simulink model "AdaptiveControl_jointSpace_AfterRedunElimi_1"  (R2020a)
settings: Solver=FixedStepDiscrete  StartTime=0.0  StopTime=Inf  FixedStep=0.001  RelTol=1e-3  EnableMultiTasking=on
values from neighbouring files (symbols this model uses):
  qr = [0 9.85590088848e-08 3.94236035539e-07 8.87031079963e-07 1.57694414216e-06 2.46397522212e-06 3.54812431985e-06 4.82939143535e-06 6.30777656863e-06 7.98327971967e-06 9.85590088848e-06 1.19256400751e-05 ... (188496 elements, 62832x3)]    [qr_62s.mat]
undefined symbols (not defined in the file or in its folder): DiscIntNeverNeededParam
libraries: slrealtimeethercatlib x27
settings Model: xpc_rtwmakecfg_data=_xpcethercatlib_  SimulationMode=external  Creator=hung  LastModifiedBy=Hung
settings SolverCC: ConcurrentTasks=on  AutoInsertRateTranBlk=on  InsertRTBMode=Never (minimum delay)
settings DataIOCC: SaveFormat=StructureWithTime  SaveState=on  SignalLoggingName=logsOut
settings OptimizationCC: BlockReduction=off  BooleanDataType=off  OptimizeBlockIOStorage=off  BufferReuse=off  GlobalBufferReuse=off  ExpressionFolding=off  LocalBlockOutputs=off  InitFltsAndDblsToZero=on  OptimizeDataStoreBuffers=off  BusAssignmentInplaceUpdate=off
settings DebuggingCC: SaveWithParameterizedLinksMsg=none  UnderspecifiedInitializationDetection=Classic  MergeDetectMultiDrivingBlocksExec=none  CheckExecutionContextPreStartOutputMsg=on  SignalResolutionControl=TryResolveAllWithWarning  SFUnexpectedBacktrackingDiag=warning  SFNoUnconditionalDefaultTransitionDiag=warning  SFExecutionAtInitializationDiag=none  UnderSpecifiedDimensionMsg=warning  ArithmeticOperatorsInVariantConditions=warning
settings HardwareCC: ProdBitPerPointer=32  ProdBitPerSizeT=32  ProdBitPerPtrDiffT=32  ProdLargestAtomicFloat=None  ProdWordSize=32  ProdLongLongMode=on  ProdHWDeviceType=Generic->32-bit x86 compatible
settings ModelReferenceCC: PropagateSignalLabelsOutOfModel=off
settings SFSimCC: SimUseLocalCustomCode=off
settings RTWCC: Description=Simulink Real-Time  SystemTargetFile=slrt.tlc  TemplateMakefile=slrt_default_tmf  RTWUseLocalCustomCode=off  CodeExecutionProfiling=on  RTWCompilerOptimization=on
settings CodeAppCC: StateflowObjectComments=on
settings SimulinkRealTimeCC: SupportVariableSizeSignals=on  RL32LogTETModifier=off  xPCConcurrentTasks=on
settings ConfigComp: CovMetricSettings=dw  CovSaveCumulativeToWorkspaceVar=on  CovSaveSingleToWorkspaceVar=on  CovExternalEMLEnable=off  CovSFcnEnable=off

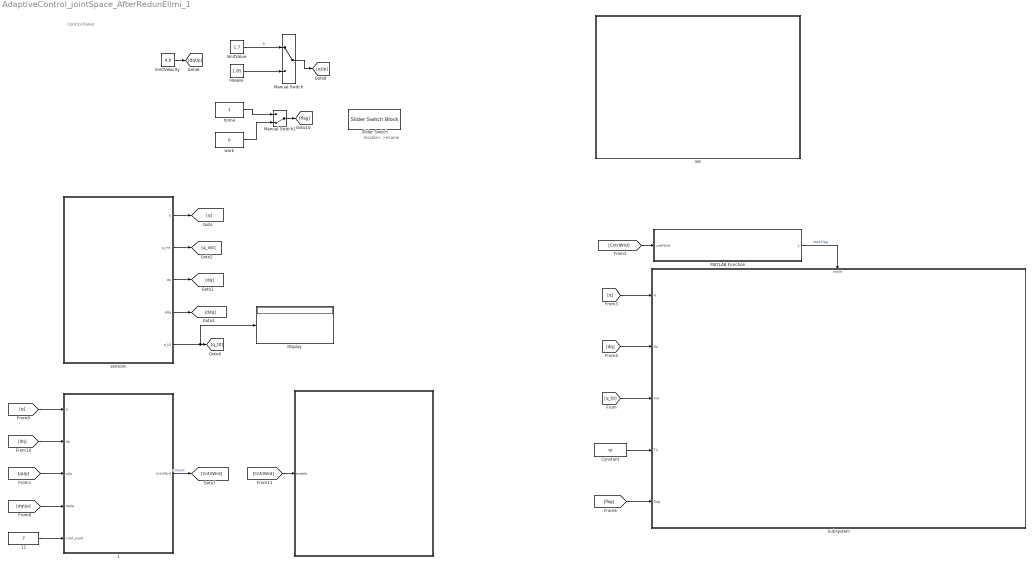
== system AdaptiveControl_jointSpace_AfterRedunElimi_1 ==
  note: Control Panel
  note: disable< >enable
  "  " : Subsystem
  1 : MATLAB Function  TreatAsAtomicUnit=on
  11 : Constant  Value=7
  Constant : Constant  Value=qr
  Display : Display
  MATLAB Function : MATLAB Function  TreatAsAtomicUnit=on
  Manual Switch : ManualSwitch
  Manual Switch1 : ManualSwitch  CurrentSetting=0
  Slider Switch : SliderSwitchBlock  LabelPosition=Hide
      settings: Values={{'Off', 'On'}, [7 15]}
  Subsystem : Subsystem
  home : Constant
  init : Subsystem
  limitValue : Constant  Value=1.7
  limitVelocity : Constant  Value=4.0
  release : Constant  Value=1.85
  sensore : Subsystem
  work : Constant  Value=0
  wires:
  ? -> ?
  sensore/1(q) -> [q]
  sensore/2(q_init) -> [q_init]
  sensore/3(dq) -> [dq]
  sensore/4(ddq) -> [ddq]
  1/1(CntrlWrd) -> [CntrlWrd]  "cntwrd"
  11/1 -> 1/5(cntrl_word)
  [dq] -> 1/2(dq)
  [q] -> 1/1(q)
  [CntrlWrd] -> "  "/1(enable)
  [qUp] -> 1/3(qUp)
  [dqUp] -> 1/4(dqUp)
  limitVelocity/1 -> [dqUp]
  limitValue/1 -> Manual Switch/1  "9"
  release/1 -> Manual Switch/2
  Manual Switch/1 -> [qUp]
  MATLAB Function/1(y) -> Subsystem/Enable  "startFlag"
  [CntrlWrd] -> MATLAB Function/1(cntrlWrd)
  sensore/5(q_t0) -> Display/1, [q_t0]
  Constant/1 -> Subsystem/4(Trj)
  work/1 -> Manual Switch1/2
  home/1 -> Manual Switch1/1
  [flag] -> Subsystem/5(flag)
  Manual Switch1/1 -> [flag]
  [q_t0] -> Subsystem/3(In3)
  [q] -> Subsystem/1(q)
  [dq] -> Subsystem/2(dq)

== system AdaptiveControl_jointSpace_AfterRedunElimi_1/   ==
  note: Contrword_setting
  enable : Inport
  Data Type Conversion : DataTypeConversion  OutDataTypeStr=uint16
  Enabled Subsystem : Subsystem  TreatAsAtomicUnit=on
  Step1 : Step  Time=5.5  SampleTime=0
  controlword_transmit : Subsystem
  wires:
  enable/1 -> Enabled Subsystem/1(In1)
  Step1/1 -> Enabled Subsystem/Enable
  Enabled Subsystem/1(ctrword) -> Data Type Conversion/1  "contrlw"
  Data Type Conversion/1 -> controlword_transmit/1(In2), controlword_transmit/2(In4), controlword_transmit/3(In6)

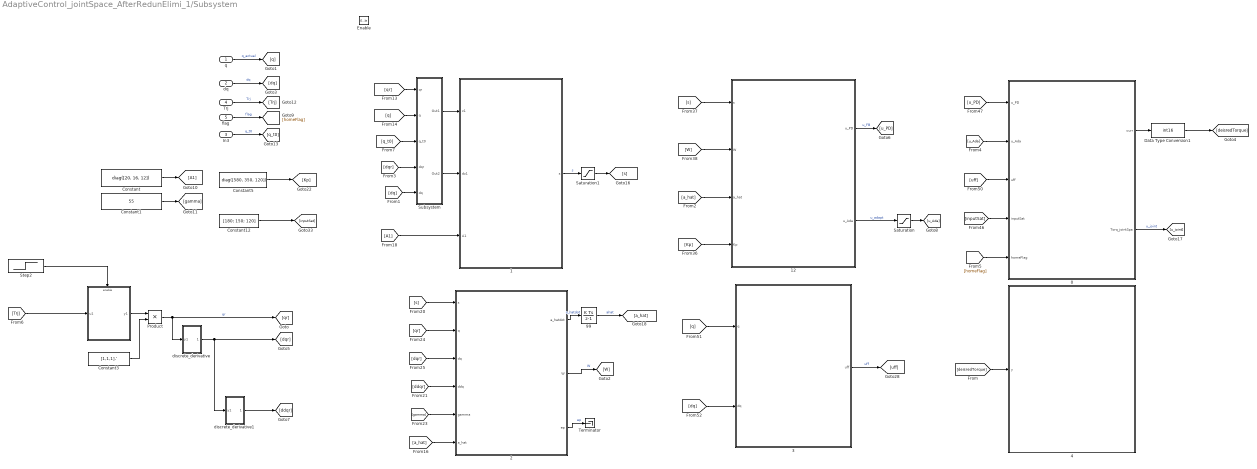
== system AdaptiveControl_jointSpace_AfterRedunElimi_1/Subsystem ==
  q : Inport
  dq : Inport  Port=2
  In3 : Inport  Port=3
  Trj : Inport  Port=4
  flag : Inport  Port=5
  Enable : EnablePort
  " " : Subsystem  TreatAsAtomicUnit=on
  0 : MATLAB Function  TreatAsAtomicUnit=on
  1 : MATLAB Function  TreatAsAtomicUnit=on
  12 : MATLAB Function  TreatAsAtomicUnit=on
  2 : MATLAB Function  TreatAsAtomicUnit=on
  3 : MATLAB Function  TreatAsAtomicUnit=on
  4 : Subsystem
  99 : DiscreteIntegrator  InitialCondition=zeros(12,1)  SampleTime=-1  ICPrevOutput=DiscIntNeverNeededParam  ICPrevScaledInput=DiscIntNeverNeededParam
  Constant : Constant  Value=diag([20, 16, 12])  VectorParams1D=off
  Constant1 : Constant  Value=55  VectorParams1D=off
  Constant12 : Constant  Value=[180; 150; 120]  VectorParams1D=off
  Constant3 : Constant  Value=[1,1,1].'  VectorParams1D=off
  Constant5 : Constant  Value=diag([580, 350, 120])  VectorParams1D=off
  Data Type Conversion1 : DataTypeConversion  OutDataTypeStr=int16
  Product : Product
  Saturation : Saturate  UpperLimit=180  LowerLimit=-180
  Saturation1 : Saturate  UpperLimit=1  LowerLimit=-1
  Step2 : Step  Time=2  SampleTime=0
  Subsystem : Subsystem
  Terminator : Terminator
  discrete_derivative : Subsystem
  discrete_derivative1 : Subsystem
  wires:
  Constant1/1 -> [gamma]
  2/1(a_hatdot) -> 99/1  "a_hatdot"
  Constant/1 -> [A1]
  [s] -> 12/1(s)
  [gamma] -> 2/5(gamma)
  0/1(curr) -> Data Type Conversion1/1
  [ddqr] -> 2/4(ddq)
  Data Type Conversion1/1 -> [deisredTorque]
  [qr] -> 2/2(q)
  [W] -> 12/2(W)
  [inputSat] -> 0/4(inputSat)
  [u_PD] -> 0/1(u_PD)
  3/1(uff) -> [uff]  "uff"
  [dqr] -> 2/3(dq)
  Constant5/1 -> [Kp]
  [Kp] -> 12/4(Kp)
  Constant12/1 -> [inputSat]
  [dq] -> 3/2(dq)
  1/1(s) -> Saturation1/1  "s"
  [A1] -> 1/3(A1)
  [q] -> 3/1(q)
  [deisredTorque] -> 4/1(y)
  q/1 -> [q]  "q_actual"
  dq/1 -> [dq]  "dq"
  [q] -> Subsystem/2(q)
  Subsystem/1(Out1) -> 1/1(z1)
  Subsystem/2(Out2) -> 1/2(dz1)
  99/1 -> [a_hat]  "ahat"
  [dq] -> Subsystem/5(dq)
  0/2(Torq_jointSpa) -> [u_joint]  "u_joint"
  2/2(W) -> [W]  "W"
  [a_hat] -> 12/3(a_hat)
  [uff] -> 0/3(uff)
  Product/1 -> discrete_derivative/1(y1), [qr]  "qr"
  Step2/1 -> " "/Enable
  [dqr] -> Subsystem/4(dqr)
  discrete_derivative/1(Out1) -> discrete_derivative1/1(y1), [dqr]
  discrete_derivative1/1(Out1) -> [ddqr]
  [qr] -> Subsystem/1(qr)
  12/1(u_PD) -> [u_PD]  "u_FB"
  12/2(u_Ada) -> Saturation/1  "u_adapt"
  [u_Ada] -> 0/2(u_Ada)
  [homeFlag] -> 0/5(homeFlag)
  Trj/1 -> [Trj]  "Trj"
  flag/1 -> [homeFlag]  "flag"
  In3/1 -> [q_t0]  "q_t0"
  [q_t0] -> Subsystem/3(q_t0)
  [a_hat] -> 2/6(a_hat)
  2/3(ep) -> Terminator/1  "ep"
  [Trj] -> " "/1(u1)
  " "/1(y1) -> Product/1
  Constant3/1 -> Product/2
  Saturation/1 -> [u_Ada]
  [s] -> 2/1(s)
  Saturation1/1 -> [s]

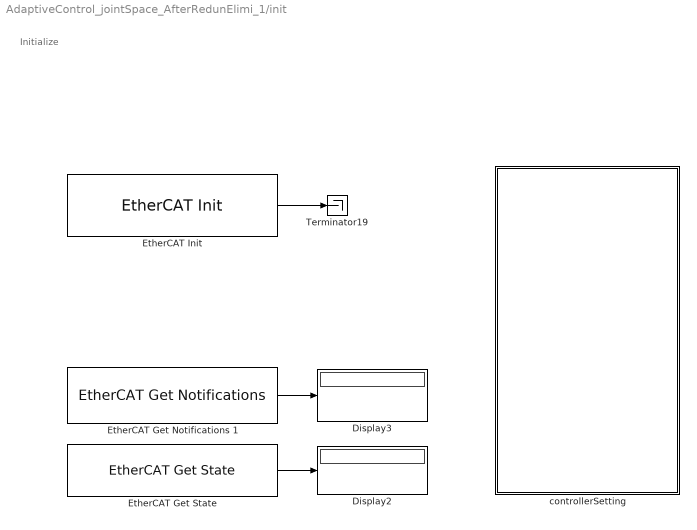
== system AdaptiveControl_jointSpace_AfterRedunElimi_1/init ==
  note: Initialize
  Display2 : Display
      settings: Format=hex (Stored Integer)
  Display3 : Display
      settings: Format=hex (Stored Integer)
  EtherCAT Get Notifications 1 : slrealtimeethercatlib/EtherCAT Get Notifications  device_id=0  sample_time=.001
  "EtherCAT Get State  " : slrealtimeethercatlib/EtherCAT Get State  device_id=0  sample_time=0
  "EtherCAT Init " : slrealtimeethercatlib/EtherCAT Init  Priority=0  config_file=E:\hhz_SRStest\EfficientModeling_Experimment\allJioints\eni8.xml  device_id=0  pci_bus=0  pci_slot=0  pci_function=0  portnum=1  initstate=2  dctuning=0  enaDebug=0  enaDC=on  errLink=off  masterDbg=off  stateChgDbg=off  baseClock=off  masterCfg=off  logFile='c:\dbglog.txt'  sample_time=0.001000  DCMode=2
  Terminator19 : Terminator
  controllerSetting : Subsystem
  wires:
  EtherCAT Get Notifications 1/1 -> Display3/1
  "EtherCAT Get State  "/1 -> Display2/1
  "EtherCAT Init "/1 -> Terminator19/1

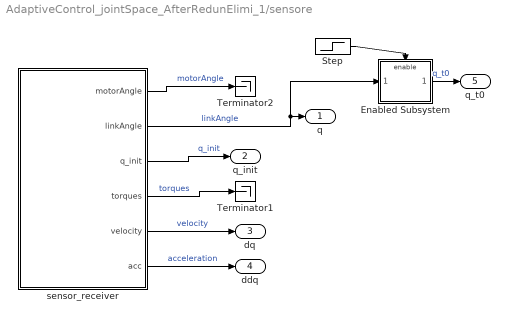
== system AdaptiveControl_jointSpace_AfterRedunElimi_1/sensore ==
  Enabled Subsystem : Subsystem  TreatAsAtomicUnit=on
  Step : Step  Time=6  Before=1  After=0  SampleTime=0
  Terminator1 : Terminator
  Terminator2 : Terminator
  sensor_receiver : Subsystem
  q : Outport
  q_init : Outport  Port=2
  dq : Outport  Port=3
  ddq : Outport  Port=4
  q_t0 : Outport  Port=5
  wires:
  sensor_receiver/3(q_init) -> q_init/1  "q_init"
  sensor_receiver/4(torques) -> Terminator1/1  "torques"
  sensor_receiver/1(motorAngle) -> Terminator2/1  "motorAngle"
  sensor_receiver/5(velocity) -> dq/1  "velocity"
  sensor_receiver/2(linkAngle) -> Enabled Subsystem/1(linkAngle), q/1  "linkAngle"
  sensor_receiver/6(acc) -> ddq/1  "acceleration"
  Step/1 -> Enabled Subsystem/Enable
  Enabled Subsystem/1(Out1) -> q_t0/1  "q_t0"

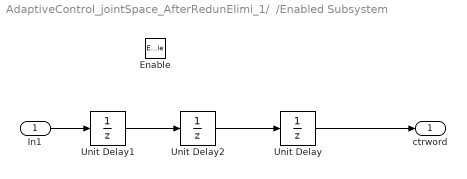
== system AdaptiveControl_jointSpace_AfterRedunElimi_1/  /Enabled Subsystem ==
  In1 : Inport
  Enable : EnablePort
  Unit Delay : UnitDelay  SampleTime=-1  HasFrameUpgradeWarning=on
  Unit Delay1 : UnitDelay  InitialCondition=7  SampleTime=-1  HasFrameUpgradeWarning=on
  Unit Delay2 : UnitDelay  InitialCondition=6  SampleTime=-1  HasFrameUpgradeWarning=on
  ctrword : Outport
  wires:
  In1/1 -> Unit Delay1/1
  Unit Delay1/1 -> Unit Delay2/1
  Unit Delay2/1 -> Unit Delay/1
  Unit Delay/1 -> ctrword/1

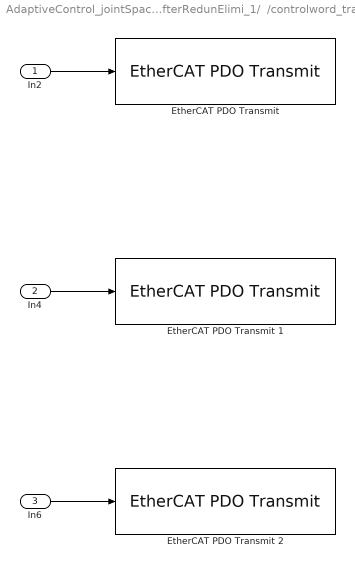
== system AdaptiveControl_jointSpace_AfterRedunElimi_1/  /controlword_transmit ==
  In2 : Inport
  In4 : Inport  Port=2
  In6 : Inport  Port=3
  "EtherCAT PDO Transmit " : slrealtimeethercatlib/EtherCAT PDO Transmit  Priority=3  sig_name=Slave_1002 [Elmo Drive ].Outputs.ControlWord  sig_offset=144  sig_type=uint16  type_size=16  sig_dim=1  device_id=0  sample_time=0.001000
  EtherCAT PDO Transmit 1 : slrealtimeethercatlib/EtherCAT PDO Transmit  Priority=3  sig_name=Slave_1004 [Elmo Drive ].Outputs.ControlWord  sig_offset=432  sig_type=uint16  type_size=16  sig_dim=1  device_id=0  sample_time=0.001000
  EtherCAT PDO Transmit 2 : slrealtimeethercatlib/EtherCAT PDO Transmit  Priority=3  sig_name=Slave_1006 [Elmo Drive ].Outputs.ControlWord  sig_offset=720  sig_type=uint16  type_size=16  sig_dim=1  device_id=0  sample_time=0.001000
  wires:
  In4/1 -> EtherCAT PDO Transmit 1/1
  In2/1 -> "EtherCAT PDO Transmit "/1
  In6/1 -> EtherCAT PDO Transmit 2/1

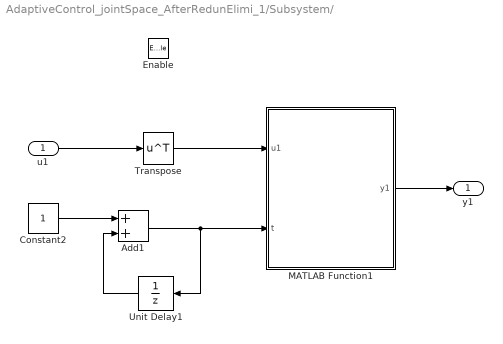
== system AdaptiveControl_jointSpace_AfterRedunElimi_1/Subsystem/  ==
  u1 : Inport
  Enable : EnablePort  StatesWhenEnabling=reset
  Add1 : Sum
  Constant2 : Constant
  MATLAB Function1 : MATLAB Function  TreatAsAtomicUnit=on
  Transpose : Math  Operator=transpose  SaturateOnIntegerOverflow=on
  Unit Delay1 : UnitDelay  SampleTime=-1  HasFrameUpgradeWarning=on
  y1 : Outport
  wires:
  MATLAB Function1/1(y1) -> y1/1
  Constant2/1 -> Add1/1
  Unit Delay1/1 -> Add1/2
  u1/1 -> Transpose/1
  Add1/1 -> Unit Delay1/1, MATLAB Function1/2(t)
  Transpose/1 -> MATLAB Function1/1(u1)

== system AdaptiveControl_jointSpace_AfterRedunElimi_1/Subsystem/4 ==
  y : Inport
  Demux : Demux  Outputs=3
  transmit : Subsystem
  wires:
  y/1 -> Demux/1
  Demux/3 -> transmit/3(theta6)
  Demux/2 -> transmit/2(theta4)
  Demux/1 -> transmit/1(theta2)

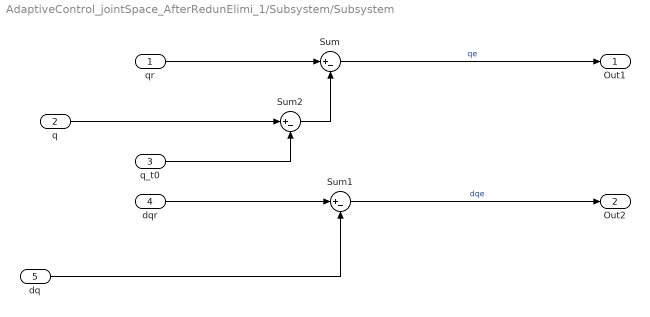
== system AdaptiveControl_jointSpace_AfterRedunElimi_1/Subsystem/Subsystem ==
  qr : Inport
  q : Inport  Port=2
  q_t0 : Inport  Port=3
  dqr : Inport  Port=4
  dq : Inport  Port=5
  Sum : Sum  Inputs=|+-
  Sum1 : Sum  Inputs=|+-
  Sum2 : Sum  Inputs=|+-
  Out1 : Outport
  Out2 : Outport  Port=2
  wires:
  qr/1 -> Sum/1
  Sum/1 -> Out1/1  "qe"
  dqr/1 -> Sum1/1
  dq/1 -> Sum1/2
  Sum1/1 -> Out2/1  "dqe"
  q/1 -> Sum2/1
  Sum2/1 -> Sum/2
  q_t0/1 -> Sum2/2

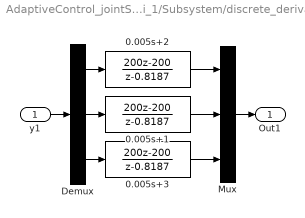
== system AdaptiveControl_jointSpace_AfterRedunElimi_1/Subsystem/discrete_derivative ==
  y1 : Inport
  0.005s+1 : DiscreteTransferFcn  Numerator=[200, -200]  Denominator=[1 -0.8187]
  0.005s+2 : DiscreteTransferFcn  Numerator=[200, -200]  Denominator=[1 -0.8187]
  0.005s+3 : DiscreteTransferFcn  Numerator=[200, -200]  Denominator=[1 -0.8187]
  Demux : Demux  Outputs=3
  Mux : Mux  Inputs=3
  Out1 : Outport
  wires:
  0.005s+1/1 -> Mux/2
  Mux/1 -> Out1/1
  Demux/2 -> 0.005s+1/1
  y1/1 -> Demux/1
  0.005s+2/1 -> Mux/1
  Demux/1 -> 0.005s+2/1
  0.005s+3/1 -> Mux/3
  Demux/3 -> 0.005s+3/1

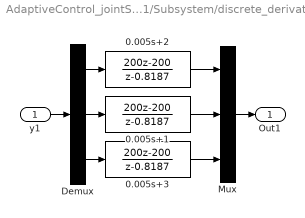
== system AdaptiveControl_jointSpace_AfterRedunElimi_1/Subsystem/discrete_derivative1 ==
  y1 : Inport
  0.005s+1 : DiscreteTransferFcn  Numerator=[200, -200]  Denominator=[1 -0.8187]
  0.005s+2 : DiscreteTransferFcn  Numerator=[200, -200]  Denominator=[1 -0.8187]
  0.005s+3 : DiscreteTransferFcn  Numerator=[200, -200]  Denominator=[1 -0.8187]
  Demux : Demux  Outputs=3
  Mux : Mux  Inputs=3
  Out1 : Outport
  wires:
  0.005s+1/1 -> Mux/2
  Mux/1 -> Out1/1
  Demux/2 -> 0.005s+1/1
  y1/1 -> Demux/1
  0.005s+2/1 -> Mux/1
  Demux/1 -> 0.005s+2/1
  0.005s+3/1 -> Mux/3
  Demux/3 -> 0.005s+3/1

== system AdaptiveControl_jointSpace_AfterRedunElimi_1/init/controllerSetting ==
  Data Type Conversion2 : DataTypeConversion  OutDataTypeStr=int8
  change_mode : Step  Time=5.3  After=10  SampleTime=0
  contr_loop_Mode : Subsystem
  wires:
  change_mode/1 -> Data Type Conversion2/1
  Data Type Conversion2/1 -> contr_loop_Mode/1(In1)

== system AdaptiveControl_jointSpace_AfterRedunElimi_1/sensore/Enabled Subsystem ==
  linkAngle : Inport
  Enable : EnablePort
  Out1 : Outport
  wires:
  linkAngle/1 -> Out1/1

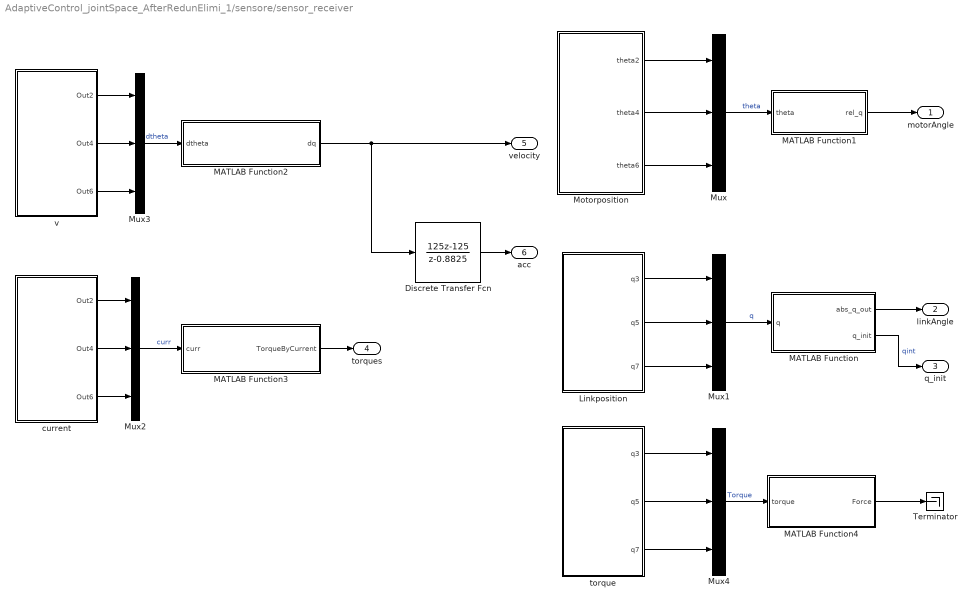
== system AdaptiveControl_jointSpace_AfterRedunElimi_1/sensore/sensor_receiver ==
  Discrete Transfer Fcn : DiscreteTransferFcn  Numerator=[125 -125]  Denominator=[1 -0.8825]
  Linkposition : Subsystem
  MATLAB Function : MATLAB Function  TreatAsAtomicUnit=on
  MATLAB Function1 : MATLAB Function  TreatAsAtomicUnit=on
  MATLAB Function2 : MATLAB Function  TreatAsAtomicUnit=on
  MATLAB Function3 : MATLAB Function  TreatAsAtomicUnit=on
  MATLAB Function4 : MATLAB Function  TreatAsAtomicUnit=on
  Motorposition : Subsystem
  Mux{,1..4} (5 alike) : Mux  Inputs=3
  Terminator : Terminator
  current : Subsystem
  torque : Subsystem
  v : Subsystem
  motorAngle : Outport
  linkAngle : Outport  Port=2
  q_init : Outport  Port=3
  torques : Outport  Port=4
  velocity : Outport  Port=5
  acc : Outport  Port=6
  wires:
  Mux/1 -> MATLAB Function1/1(theta)  "theta"
  MATLAB Function/2(q_init) -> q_init/1  "qint"
  Mux1/1 -> MATLAB Function/1(q)  "q"
  Mux3/1 -> MATLAB Function2/1(dtheta)  "dtheta"
  Linkposition/1(q3) -> Mux1/1
  Linkposition/2(q5) -> Mux1/2
  Linkposition/3(q7) -> Mux1/3
  Motorposition/1(theta2) -> Mux/1
  Motorposition/3(theta6) -> Mux/3
  Motorposition/2(theta4) -> Mux/2
  v/1(Out2) -> Mux3/1
  v/2(Out4) -> Mux3/2
  v/3(Out6) -> Mux3/3
  current/1(Out2) -> Mux2/1
  current/2(Out4) -> Mux2/2
  current/3(Out6) -> Mux2/3
  Mux2/1 -> MATLAB Function3/1(curr)  "curr"
  torque/3(q7) -> Mux4/3
  torque/1(q3) -> Mux4/1
  torque/2(q5) -> Mux4/2
  Mux4/1 -> MATLAB Function4/1(torque)  "Torque"
  MATLAB Function/1(abs_q_out) -> linkAngle/1
  MATLAB Function1/1(rel_q) -> motorAngle/1
  MATLAB Function3/1(TorqueByCurrent) -> torques/1
  MATLAB Function4/1(Force) -> Terminator/1
  Discrete Transfer Fcn/1 -> acc/1
  MATLAB Function2/1(dq) -> Discrete Transfer Fcn/1, velocity/1

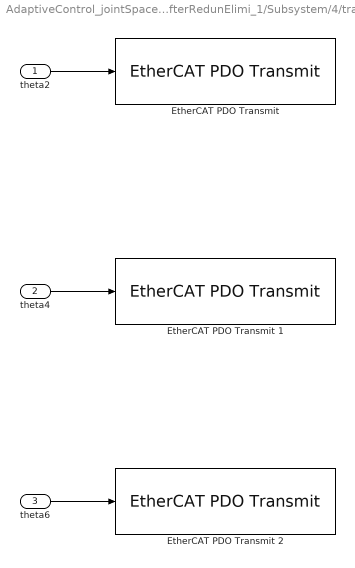
== system AdaptiveControl_jointSpace_AfterRedunElimi_1/Subsystem/4/transmit ==
  theta2 : Inport
  theta4 : Inport  Port=2
  theta6 : Inport  Port=3
  "EtherCAT PDO Transmit " : slrealtimeethercatlib/EtherCAT PDO Transmit  Priority=3  sig_name=Slave_1002 [Elmo Drive ].Outputs.TargetTorque  sig_offset=176  sig_type=int16  type_size=16  sig_dim=1  device_id=0  sample_time=0.001000
  EtherCAT PDO Transmit 1 : slrealtimeethercatlib/EtherCAT PDO Transmit  Priority=3  sig_name=Slave_1004 [Elmo Drive ].Outputs.TargetTorque  sig_offset=464  sig_type=int16  type_size=16  sig_dim=1  device_id=0  sample_time=0.001000
  EtherCAT PDO Transmit 2 : slrealtimeethercatlib/EtherCAT PDO Transmit  Priority=3  sig_name=Slave_1006 [Elmo Drive ].Outputs.TargetTorque  sig_offset=752  sig_type=int16  type_size=16  sig_dim=1  device_id=0  sample_time=0.001000
  wires:
  theta6/1 -> EtherCAT PDO Transmit 2/1
  theta2/1 -> "EtherCAT PDO Transmit "/1
  theta4/1 -> EtherCAT PDO Transmit 1/1

== system AdaptiveControl_jointSpace_AfterRedunElimi_1/init/controllerSetting/contr_loop_Mode ==
  In1 : Inport
  "EtherCAT PDO Transmit " : slrealtimeethercatlib/EtherCAT PDO Transmit  Priority=3  sig_name=Slave_1002 [Elmo Drive ].Outputs.ModeOfOperation  sig_offset=160  sig_type=int8  type_size=8  sig_dim=1  device_id=0  sample_time=0.001000
  EtherCAT PDO Transmit 1 : slrealtimeethercatlib/EtherCAT PDO Transmit  Priority=3  sig_name=Slave_1004 [Elmo Drive ].Outputs.ModeOfOperation  sig_offset=448  sig_type=int8  type_size=8  sig_dim=1  device_id=0  sample_time=0.001000
  EtherCAT PDO Transmit 2 : slrealtimeethercatlib/EtherCAT PDO Transmit  Priority=3  sig_name=Slave_1006 [Elmo Drive ].Outputs.ModeOfOperation  sig_offset=736  sig_type=int8  type_size=8  sig_dim=1  device_id=0  sample_time=0.001000
  wires:
  In1/1 -> EtherCAT PDO Transmit 2/1, EtherCAT PDO Transmit 1/1, "EtherCAT PDO Transmit "/1

== system AdaptiveControl_jointSpace_AfterRedunElimi_1/sensore/sensor_receiver/Linkposition ==
  EtherCAT PDO Receive : slrealtimeethercatlib/EtherCAT PDO Receive  Priority=2  sig_name=Slave_1003 [Elmo Drive ].Inputs.ActualPosition  sig_offset=400  sig_type=int32  type_size=32  sig_dim=1  device_id=0  sample_time=0.001000
  EtherCAT PDO Receive1 : slrealtimeethercatlib/EtherCAT PDO Receive  Priority=2  sig_name=Slave_1005 [Elmo Drive ].Inputs.ActualPosition  sig_offset=688  sig_type=int32  type_size=32  sig_dim=1  device_id=0  sample_time=0.001000
  EtherCAT PDO Receive2 : slrealtimeethercatlib/EtherCAT PDO Receive  Priority=2  sig_name=Slave_1007 [Elmo Drive ].Inputs.ActualPosition  sig_offset=976  sig_type=int32  type_size=32  sig_dim=1  device_id=0  sample_time=0.001000
  q3 : Outport
  q5 : Outport  Port=2
  q7 : Outport  Port=3
  wires:
  EtherCAT PDO Receive/1 -> q3/1
  EtherCAT PDO Receive1/1 -> q5/1
  EtherCAT PDO Receive2/1 -> q7/1

== system AdaptiveControl_jointSpace_AfterRedunElimi_1/sensore/sensor_receiver/Motorposition ==
  EtherCAT PDO Receive : slrealtimeethercatlib/EtherCAT PDO Receive  Priority=2  sig_name=Slave_1002 [Elmo Drive ].Inputs.MotorPosition  sig_offset=160  sig_type=int32  type_size=32  sig_dim=1  device_id=0  sample_time=0.001000
  EtherCAT PDO Receive1 : slrealtimeethercatlib/EtherCAT PDO Receive  Priority=2  sig_name=Slave_1004 [Elmo Drive ].Inputs.MotorPosition  sig_offset=448  sig_type=int32  type_size=32  sig_dim=1  device_id=0  sample_time=0.001000
  EtherCAT PDO Receive2 : slrealtimeethercatlib/EtherCAT PDO Receive  Priority=2  sig_name=Slave_1006 [Elmo Drive ].Inputs.MotorPosition  sig_offset=736  sig_type=int32  type_size=32  sig_dim=1  device_id=0  sample_time=0.001000
  theta2 : Outport
  theta4 : Outport  Port=2
  theta6 : Outport  Port=3
  wires:
  EtherCAT PDO Receive1/1 -> theta4/1
  EtherCAT PDO Receive/1 -> theta2/1
  EtherCAT PDO Receive2/1 -> theta6/1

== system AdaptiveControl_jointSpace_AfterRedunElimi_1/sensore/sensor_receiver/current ==
  EtherCAT PDO Receive : slrealtimeethercatlib/EtherCAT PDO Receive  Priority=2  sig_name=Slave_1002 [Elmo Drive ].Inputs.ActualCurrent  sig_offset=224  sig_type=int16  type_size=16  sig_dim=1  device_id=0  sample_time=0.001000
  EtherCAT PDO Receive1 : slrealtimeethercatlib/EtherCAT PDO Receive  Priority=2  sig_name=Slave_1004 [Elmo Drive ].Inputs.ActualCurrent  sig_offset=512  sig_type=int16  type_size=16  sig_dim=1  device_id=0  sample_time=0.001000
  EtherCAT PDO Receive2 : slrealtimeethercatlib/EtherCAT PDO Receive  Priority=2  sig_name=Slave_1006 [Elmo Drive ].Inputs.ActualCurrent  sig_offset=800  sig_type=int16  type_size=16  sig_dim=1  device_id=0  sample_time=0.001000
  Out2 : Outport
  Out4 : Outport  Port=2
  Out6 : Outport  Port=3
  wires:
  EtherCAT PDO Receive2/1 -> Out6/1
  EtherCAT PDO Receive/1 -> Out2/1
  EtherCAT PDO Receive1/1 -> Out4/1

== system AdaptiveControl_jointSpace_AfterRedunElimi_1/sensore/sensor_receiver/torque ==
  EtherCAT PDO Receive : slrealtimeethercatlib/EtherCAT PDO Receive  Priority=2  sig_name=Slave_1003 [Elmo Drive ].Inputs.ActualTorque  sig_offset=384  sig_type=int16  type_size=16  sig_dim=1  device_id=0  sample_time=0.001000
  EtherCAT PDO Receive1 : slrealtimeethercatlib/EtherCAT PDO Receive  Priority=2  sig_name=Slave_1005 [Elmo Drive ].Inputs.ActualTorque  sig_offset=672  sig_type=int16  type_size=16  sig_dim=1  device_id=0  sample_time=0.001000
  EtherCAT PDO Receive2 : slrealtimeethercatlib/EtherCAT PDO Receive  Priority=2  sig_name=Slave_1007 [Elmo Drive ].Inputs.ActualTorque  sig_offset=960  sig_type=int16  type_size=16  sig_dim=1  device_id=0  sample_time=0.001000
  q3 : Outport
  q5 : Outport  Port=2
  q7 : Outport  Port=3
  wires:
  EtherCAT PDO Receive/1 -> q3/1
  EtherCAT PDO Receive1/1 -> q5/1
  EtherCAT PDO Receive2/1 -> q7/1

== system AdaptiveControl_jointSpace_AfterRedunElimi_1/sensore/sensor_receiver/v ==
  EtherCAT PDO Receive : slrealtimeethercatlib/EtherCAT PDO Receive  Priority=2  sig_name=Slave_1002 [Elmo Drive ].Inputs.MotorVelocity  sig_offset=192  sig_type=int32  type_size=32  sig_dim=1  device_id=0  sample_time=0.001000
  EtherCAT PDO Receive1 : slrealtimeethercatlib/EtherCAT PDO Receive  Priority=2  sig_name=Slave_1004 [Elmo Drive ].Inputs.MotorVelocity  sig_offset=480  sig_type=int32  type_size=32  sig_dim=1  device_id=0  sample_time=0.001000
  EtherCAT PDO Receive2 : slrealtimeethercatlib/EtherCAT PDO Receive  Priority=2  sig_name=Slave_1006 [Elmo Drive ].Inputs.MotorVelocity  sig_offset=768  sig_type=int32  type_size=32  sig_dim=1  device_id=0  sample_time=0.001000
  Out2 : Outport
  Out4 : Outport  Port=2
  Out6 : Outport  Port=3
  wires:
  EtherCAT PDO Receive1/1 -> Out4/1
  EtherCAT PDO Receive/1 -> Out2/1
  EtherCAT PDO Receive2/1 -> Out6/1

== matlab function AdaptiveControl_jointSpace_AfterRedunElimi_1/Subsystem/0 ==
  data: u_PD input; u_Ada input; uff input; curr output; Torq_jointSpa output; inputSat input; homeFlag input
function [curr,Torq_jointSpa] = Tor2cur(u_PD,u_Ada, uff, inputSat,homeFlag)

% linkLens = linkLen(2:4);
[curr,Torq_jointSpa] = Torque2Current_JointControl(u_PD,u_Ada, uff, inputSat,homeFlag);


end

== matlab function AdaptiveControl_jointSpace_AfterRedunElimi_1/Subsystem/3 ==
  data: q input; uff output; dq input
function uff = fcn(q,dq)

uff = GravityAndFriction(q,dq);
end

== matlab function AdaptiveControl_jointSpace_AfterRedunElimi_1/Subsystem/1 ==
  data: z1 input; s output; dz1 input; A1 input
function s = biasSurface(z1,dz1,A1)

% z1 = xd - x;
% dz1 = dxd - dx;

s = dz1 + A1*z1;

end

== matlab function AdaptiveControl_jointSpace_AfterRedunElimi_1/MATLAB Function ==
  data: cntrlWrd input; y output
function y = fcn(cntrlWrd)

if cntrlWrd == 7
    y = 0;
else
    y = 1;
end
end

== matlab function AdaptiveControl_jointSpace_AfterRedunElimi_1/sensore/sensor_receiver/MATLAB Function ==
  data: q input; abs_q_out output; q_init output
function [abs_q_out,q_init] = encoder_sol(q)

[abs_q_out,q_init] = encoder_normalize(q);
end

== matlab function AdaptiveControl_jointSpace_AfterRedunElimi_1/Subsystem/ /MATLAB Function1 ==
  data: u1 input; y1 output; t input
function y1 = fcn(u1,t)
m=size(u1);
n=m(2);
if t<n
    y1=[u1(1,t);u1(2,t);u1(3,t)];
%         y1=[0;0;u1(3,t)];
%         y1=[0;u1(2,t);0];
%         y1=[u1(1,t);0;0];


else
    y1=[u1(1,n);u1(2,n);u1(3,n)];
%     y1=[0;0;u1(3,n)];
%       y1=[0;u1(2,n);0];
%       y1=[u1(1,n);0;0];

end
end

== matlab function AdaptiveControl_jointSpace_AfterRedunElimi_1/sensore/sensor_receiver/MATLAB Function1 ==
  data: theta input; rel_q output
function rel_q = fcn(theta)

rel_q = Motortheta_sol(theta);
end

== matlab function AdaptiveControl_jointSpace_AfterRedunElimi_1/sensore/sensor_receiver/MATLAB Function2 ==
  data: dtheta input; dq output
function dq = fcn(dtheta)
dq = dq_normlize(dtheta);
end

== matlab function AdaptiveControl_jointSpace_AfterRedunElimi_1/sensore/sensor_receiver/MATLAB Function3 ==
  data: curr input; TorqueByCurrent output
function TorqueByCurrent = fcn(curr)

TorqueByCurrent = Current2Torque(curr);
end

== matlab function AdaptiveControl_jointSpace_AfterRedunElimi_1/sensore/sensor_receiver/MATLAB Function4 ==
  data: torque input; Force output
function Force = fcn(torque)
Force = Force_sol(torque);
end

== matlab function AdaptiveControl_jointSpace_AfterRedunElimi_1/Subsystem/2 ==
  data: s input; a_hatdot output; q input; dq input; ddq input; gamma input; W output; a_hat input; ep output
function [a_hatdot,W,ep] = fcn(s,q,dq,ddq,gamma,a_hat)
wf1 = [sign(dq(1)),dq(1)];
wf2 = [sign(dq(2)),dq(2)];
wf3 = [sign(dq(3)),dq(3)];

Wf = blkdiag(wf1,wf2,wf3);

Wd = W_tau_After_fun(q,dq,ddq);

W = [Wd,Wf];
ep = Yu_int - Yx_int*a_hat;
if norm(s,1)<1e-4
    a_hatdot = zeros(12,1);
else
    a_hatdot = -gamma * W.' * (s.*[-1;-1;1]);
%         a_hatdot = -gamma * W.' * (s.*[-1;0;0]);
%         a_hatdot = -gamma * W.' * (s.*[0;-1;0]);
%         a_hatdot = -gamma * W.' * (s.*[0;0;1]);


end
end

== matlab function AdaptiveControl_jointSpace_AfterRedunElimi_1/1 ==
  data: q input; CntrlWrd output; dq input; qUp input; dqUp input; cntrl_word input
function CntrlWrd  = StateMechanisms(q,dq,qUp,dqUp,cntrl_word)



if cntrl_word == 15
    if JointLimit(q,dq,qUp,dqUp)==1 %
        CntrlWrd = 0x0F;
    else
        CntrlWrd = 0x07;
    end
else
        CntrlWrd = 0x07;
end

end

== matlab function AdaptiveControl_jointSpace_AfterRedunElimi_1/Subsystem/12 ==
  data: s input; W input; a_hat input; Kp input; u_PD output; u_Ada output
function [u_PD,u_Ada] = fcn(s, W, a_hat, Kp)

u_PD = Kp * s;

u_Ada = W * a_hat;

% u = u_1 + u_2;% 

end
